simulink model "dcc4"  (Simulink 3.00)
settings: Solver=ode45  SolverMode=SingleTasking  StartTime=0.0  StopTime=20  MaxStep=0.01  RelTol=1e-3  AbsTol=1e-3
settings Model: TimeSaveName=t  SaveOutput=off

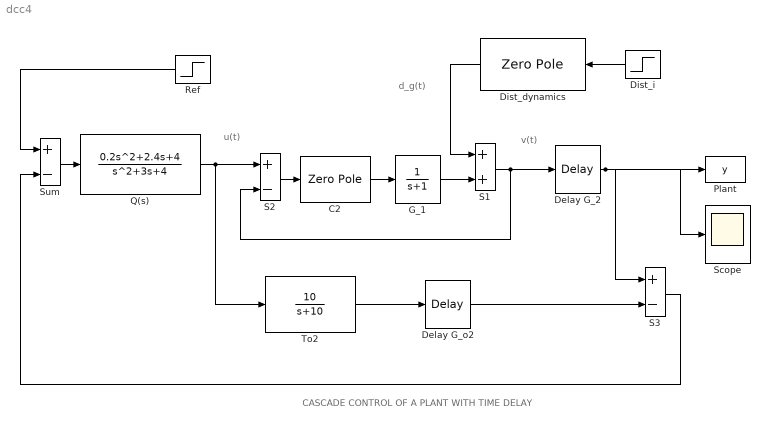
== system dcc4 ==
  note: CASCADE CONTROL OF A PLANT WITH TIME DELAY
  note: d_g(t)
  note: u(t)
  note: v(t)
  C2 : ZeroPole  Zeros=[-1]  Poles=[0]  Gain=[10]
  Delay G_2 : TransportDelay  DelayTime=2  InitialInput=0  BufferSize=4096
  Delay G_o2 : TransportDelay  DelayTime=2  InitialInput=0  BufferSize=4096
  Dist_dynamics : ZeroPole  Orientation=left  Zeros=[]  Poles=[-3;-8]  Gain=[24]
  Dist_i : Step  Orientation=left  Time=10  Before=0  After=1  SampleTime=0
  G_1 : TransferFcn  Numerator=[1]  Denominator=[1 1]
  Plant : ToWorkspace  VariableName=y  SampleTime=0  SaveFormat=Matrix
      settings: Buffer=6000
  Q(s) : TransferFcn  Numerator=[0.2 2.4 4]  Denominator=[1 3 4]
  Ref : Step  Orientation=left  Time=1  Before=0  After=1  SampleTime=0
  S1 : Sum  Inputs=++  SaturateOnIntegerOverflow=on
  S2 : Sum  Inputs=+-  SaturateOnIntegerOverflow=on
  S3 : Sum  Inputs=+-  SaturateOnIntegerOverflow=on
  Scope : Scope
      settings: TickLabels=on  TimeRange=20.000000  YMin=-1.5  YMax=1.5  SaveToWorkspace=off  SaveName=ScopeData  DataFormat=Matrix
  Sum : Sum  Inputs=+-  SaturateOnIntegerOverflow=on
  To2 : TransferFcn  Numerator=[10]  Denominator=[1 10]
  wires:
  Sum/1 -> Q(s)/1
  G_1/1 -> S1/2
  C2/1 -> G_1/1
  S2/1 -> C2/1
  Dist_i/1 -> Dist_dynamics/1
  Dist_dynamics/1 -> S1/1
  To2/1 -> Delay G_o2/1
  S3/1 -> Sum/2
  Delay G_2/1 -> Plant/1, Scope/1, S3/1
  Ref/1 -> Sum/1
  Delay G_o2/1 -> S3/2
  Q(s)/1 -> S2/1, To2/1
  S1/1 -> Delay G_2/1, S2/2
